simulink model "DT_DSM_CIFF_MODEL_SECOND_ORDER_OSR_2048_FLICKER_NOISE"  (R2025b)
settings: Solver=VariableStepAuto  StartTime=0.0  StopTime=1  RelTol=1e-3
libraries: dspobslib x2, simulink_extras x1, cstblocks x1
settings Model: Creator=Team_33  LastModifiedBy=k2vas

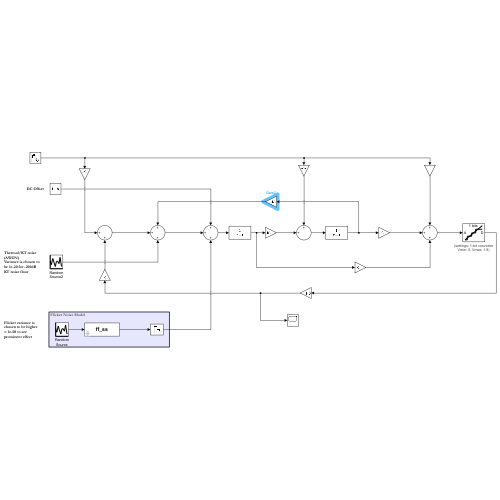
[thumbnail: Simulink's stored preview of the top-level diagram]
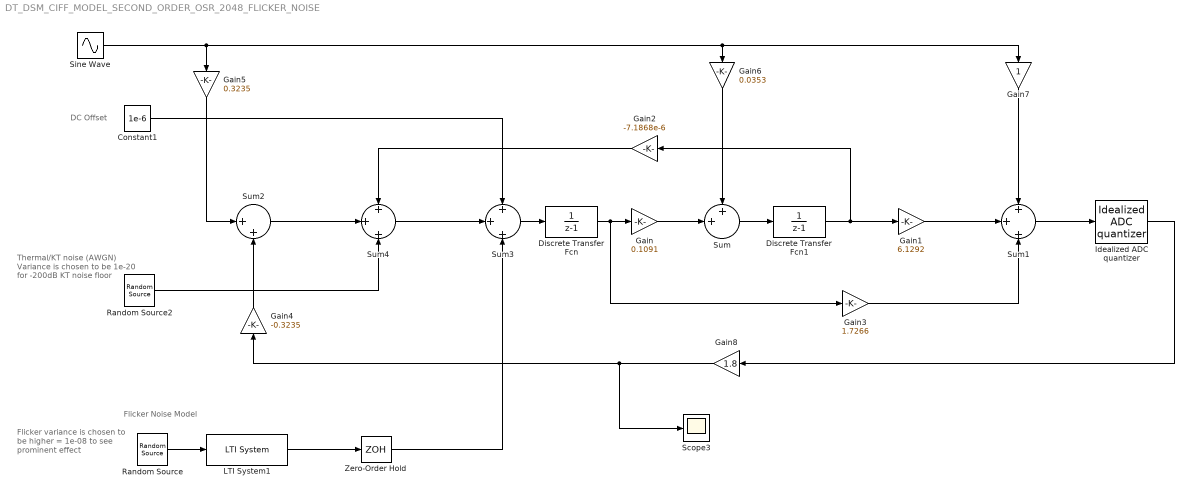
== system DT_DSM_CIFF_MODEL_SECOND_ORDER_OSR_2048_FLICKER_NOISE ==
  note: Flicker variance is
      | chosen to be higher
      | = 1e-08 to see
      | prominent effect
  note: DC Offset
  note: Thermal/KT noise
      | (AWGN)
      | Variance is chosen to
      | be 1e-20 for -200dB
      | KT noise floor
  note: Flicker Noise Model
  Constant1 : Constant  Value=1e-6
  Discrete Transfer Fcn : DiscreteTransferFcn  Denominator=[1 -1]
  Discrete Transfer Fcn1 : DiscreteTransferFcn  Denominator=[1 -1]
  Gain : Gain  Gain=0.1091
  Gain1 : Gain  Gain=6.1292
  Gain2 : Gain  Gain=-7.1868e-6
  Gain3 : Gain  Gain=1.7266
  Gain4 : Gain  Gain=-0.3235
  Gain5 : Gain  Gain=0.3235
  Gain6 : Gain  Gain=0.0353
  Gain7 : Gain
  Gain8 : Gain  Gain=1.8
  Idealized ADC quantizer : simulink_extras/Additional Discrete/Idealized ADC quantizer  NumberOfConverterBits=1  Vmin=0  Vmax=1.8  OutputDataType=int16  OutputNegativeValues=off
  LTI System1 : cstblocks/LTI System  sys=ff_ss  IC=[]  PadeOrder=0
  Random Source : dspobslib/Random Source  SrcType=Gaussian  NormMethod=Ziggurat  CltLength=12  MinVal=0  MaxVal=1  MeanVal=0  VarVal=1e-10  RepMode=Not repeatable  rawSeed=1  IsInherit=off  SampMode=Discrete  SampTime=1/(2000*2048)  SampFrame=1  DataType=Double  OutComplex=Real  OutputFrames=off
  Random Source2 : dspobslib/Random Source  SrcType=Gaussian  NormMethod=Ziggurat  CltLength=12  MinVal=0  MaxVal=1  MeanVal=0  VarVal=1e-20  RepMode=Not repeatable  rawSeed=1  IsInherit=off  SampMode=Discrete  SampTime=1/(2000*2048)  SampFrame=1  DataType=Double  OutComplex=Real  OutputFrames=off
  Scope3 : Scope
      settings: ActiveDisplayYMinimum=1.03994  ActiveDisplayYMaximum=1.04051  DataLoggingVariableName=output_data  DataLoggingSaveFormat=Array
  Sine Wave : Sin  Amplitude=0.5  Bias=0.9  Frequency=(2000*2048)*(2*pi*127)/(32768*32)  SampleTime=1/(2000*2048)
  Sum : Sum  Inputs=++|
  Sum1 : Sum  Inputs=+|+|+
  Sum2 : Sum  Inputs=|++
  Sum3 : Sum  Inputs=+|+|+
  Sum4 : Sum  Inputs=+|+|+
  Zero-Order Hold : ZeroOrderHold  SampleTime=1/(2000*2048)
  wires:
  Gain/1 -> Sum/2
  Gain7/1 -> Sum1/1
  Gain1/1 -> Sum1/2
  Discrete Transfer Fcn1/1 -> Gain2/1, Gain1/1
  Gain6/1 -> Sum/1
  Sine Wave/1 -> Gain7/1, Gain6/1, Gain5/1
  Sum/1 -> Discrete Transfer Fcn1/1
  Gain3/1 -> Sum1/3
  Gain4/1 -> Sum2/2
  Sum1/1 -> Idealized ADC quantizer/1
  Discrete Transfer Fcn/1 -> Gain/1, Gain3/1
  Idealized ADC quantizer/1 -> Gain8/1
  LTI System1/1 -> Zero-Order Hold/1
  Random Source/1 -> LTI System1/1
  Sum3/1 -> Discrete Transfer Fcn/1
  Zero-Order Hold/1 -> Sum3/3
  Gain8/1 -> Scope3/1, Gain4/1
  Constant1/1 -> Sum3/1
  Sum4/1 -> Sum3/2
  Random Source2/1 -> Sum4/3
  Sum2/1 -> Sum4/2
  Gain2/1 -> Sum4/1
  Gain5/1 -> Sum2/1
